simulink library "Roof"  (R2018b)
settings: Solver=ode45  StartTime=0.0  StopTime=10.0  RelTol=1e-3  EnableMultiTasking=on
libraries: carnot x3
settings Model: Creator=lena.frank  LastModifiedBy=P41573
settings DataIOCC: LimitDataPoints=on  SaveFormat=Array  SignalLoggingSaveFormat=ModelDataLogs
settings OptimizationCC: ExpressionDepthLimit=2147483647  LifeSpan=inf
settings DebuggingCC: UnderspecifiedInitializationDetection=Classic  MergeDetectMultiDrivingBlocksExec=none  SolverPrmCheckMsg=warning  FcnCallInpInsideContextMsg=warning  StateNameClashWarn=warning  SFUnexpectedBacktrackingDiag=warning  SFNoUnconditionalDefaultTransitionDiag=warning  SFExecutionAtInitializationDiag=none
settings HardwareCC: ProdBitPerPointer=32  ProdBitPerSizeT=32  ProdBitPerPtrDiffT=32  ProdLargestAtomicFloat=None  ProdIntDivRoundTo=Undefined  ProdEndianess=Unspecified  ProdWordSize=32  ProdHWDeviceType=32-bit Generic
settings ModelReferenceCC: PropagateSignalLabelsOutOfModel=off
settings SFSimCC: SimUseLocalCustomCode=off
settings RTWCC: RTWUseLocalCustomCode=off
settings CodeAppCC: StateflowObjectComments=on
settings GRTTargetCC: TargetLangStandard=C89/C90 (ANSI)  GeneratePreprocessorConditionals=Disable all  CombineOutputUpdateFcns=off  GRTInterface=on
settings ConfigComp: CovMetricSettings=dw  CovHtmlReporting=on  CovSaveCumulativeToWorkspaceVar=on  CovSaveSingleToWorkspaceVar=on  CovExternalEMLEnable=off

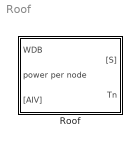
== system Roof ==
  Roof : Subsystem  mask(outer roof){wallsize=[5 5], pos=[0 0 0], t0=20, d=[0.015 0.38 0.02], cond=[1.4 0.79 0.7], cwall=[0.28 0.28 0.28]*3600, rho=[2000 1800 1400], reflectground=0.2, abs_emiss=[0.6, 0.9, 0.9], tau=1000*3600, dactive=-1}
      mask prompts: wallsize "size of wall [m] [height width]"; pos "position [inclination azimuth rotation]"; t0 "initial temperature [degree centigrade]"; d "thickness of nodes [m] (vector)"; cond "conductivity of nodes [W/(m*K)] (vector)"; cwall "capacity of nodes [J/(kg*K)] (vector)"; rho "density [kg/m^3]"; reflectground "reflection of ground"; abs_emiss "[outer absorption, outer emission, inner emisson]"; tau "time-constant of wall [s]"; dactive "depth of active layer in m from outside (-1, if none)"
      mask help:
      | This is the model of an outer roof of a house.
      | first element of the vector = layer to surrounding
      | last element of the vector = layer to room
      mask init:
      | absorption_out = min(1, max(abs_emiss(1),0));
      | nodes = length(d);
      | h = wallsize(1);
      | w = wallsize(2);
      | wallsurface = h*w;
      | emission_c = abs_emiss(3);
      | emission_out = abs_emiss(2);
      | active = 0;
      | if (dactive>=0) active=1; end
      | 
      | %für Variablen in shaderad
      | wallangle = pos(1);
      | wallazimut = pos(2);
      | wallheight=h;
      | wallwidth=w;
      mask Help: web(fullfile(path_carnot('help'),'Roof.html'),'-helpbrowser')

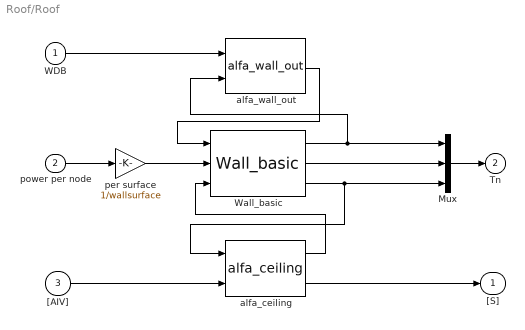
== system Roof/Roof ==
  WDB : Inport
  power per node : Inport  Port=2
  "[AIV]" : Inport  Port=3
  Mux : Mux  Inputs=3
  Wall_basic : carnot/Basic/Thermal_Models/Wall_basic  tau=tau  t0=t0  d=d  dactive=dactive  cond=cond  cwall=cwall  rho=rho
      settings: SourceProductName=Carnot
  alfa_ceiling : carnot/Basic/Heat_Transfer/alfa_ceiling  active=active  emission_c=emission_c  wallsurface=wallsurface
      settings: SourceProductName=Carnot
  alfa_wall_out : carnot/Basic/Heat_Transfer/alfa_wall_out  pos=pos  absorption_out=absorption_out  emission_out=emission_out  wallsurface=wallsurface
      settings: SourceProductName=Carnot
  per surface : Gain  Gain=1/wallsurface  SaturateOnIntegerOverflow=on  OutDataTypeStr=Inherit: Same as input  ParamDataTypeStr=Inherit: Same as input
  "[S]" : Outport
  Tn : Outport  Port=2
  wires:
  Mux/1 -> Tn/1
  alfa_wall_out/1 -> Wall_basic/1
  WDB/1 -> alfa_wall_out/1
  Wall_basic/1 -> alfa_wall_out/2, Mux/1
  Wall_basic/3 -> alfa_ceiling/1, Mux/3
  Wall_basic/2 -> Mux/2
  alfa_ceiling/1 -> Wall_basic/3
  "[AIV]"/1 -> alfa_ceiling/2
  alfa_ceiling/2 -> "[S]"/1
  power per node/1 -> per surface/1
  per surface/1 -> Wall_basic/2
